simulink model "PMSMDriveThermal"  (R2025b)
settings: Solver=ode15s  StartTime=0.0  StopTime=1  MaxStep=1e-3  MinStep=1e-10  RelTol=1e-2  AbsTol=1e-6  EnableMultiTasking=on
PreLoadFcn:
  | PMSMDriveThermalData;
values from neighbouring files (symbols this model uses):
  N = 6    [E25runs1.mat]
  PM = 0.03    [E25runs1.mat]
undefined symbols (not defined in the file or in its folder): f_losses, Isc_losses, losses_oc, losses_sc
libraries: batteryecm_lib x280, fl_lib x53, nesl_utility x21, ee_lib x10, SimscapeFluids_lib x3, eePmsmFieldOrientedControl x1
(part 1 of 24)
CloseFcn:
  | try,close(h1_PMSMDriveThermal),end
  | clear h1_PMSMDriveThermal
  | try,close(h2_PMSMDriveThermal),end
  | clear h2_PMSMDriveThermal
  | 
  | clear simlog_PMSMDriveThermal
  | clear logsout_PMSMDriveThermal
  | 
  | clear alpha alpha_flux f_losses fc fnom fsw Imax
  | clear Isc losses J L0 Ld losses_oc losses_sc Lq N
  | clear omegam_nom PM Pmax rpm_nom Rs
  | clear Rd_percent_rotor Rm_percent_rotor
  | clear rotor_thermal_mass stator_thermal_mass
  | clear Tmax Tmeas Ts Tsc Isc_losses
Description:
  | Three-Phase PMSM Drive with Thermal Model
settings Model: Creator=The MathWorks, Inc.  LastModifiedBy=muizz
settings SolverCC: AutoScaleAbsTol=off  InitialStep=1e-8  MaxConsecutiveMinStep=20  ZeroCrossAlgorithm=Adaptive  AlgebraicLoopSolver=TrustRegion  MaxZcPerStep=1.0
settings DataIOCC: LimitDataPoints=on  MaxDataPoints=690000  SaveFormat=Array  ReturnWorkspaceOutputs=off  SignalLoggingName=logsout_PMSMDriveThermal
settings OptimizationCC: ReuseModelBlockBuffer=off  LifeSpan=inf
settings DebuggingCC: UnderspecifiedInitializationDetection=Classic  MergeDetectMultiDrivingBlocksExec=none  MaxConsecutiveZCsMsg=none  IgnoredZcDiagnostic=none  UnconnectedInputMsg=warning  UnconnectedOutputMsg=warning  UnconnectedLineMsg=warning  AllowSymbolicDim=off  PregeneratedLibrarySubsystemCodeDiagnostic=none  SFUnexpectedBacktrackingDiag=warning  SFNoUnconditionalDefaultTransitionDiag=warning  SFExecutionAtInitializationDiag=none  ArithmeticOperatorsInVariantConditions=warning
settings HardwareCC: ProdBitPerPointer=32.0  ProdBitPerSizeT=32.0  ProdBitPerPtrDiffT=32.0  ProdLargestAtomicFloat=None  ProdIntDivRoundTo=Undefined  ProdEndianess=Unspecified  ProdWordSize=32.0  ProdHWDeviceType=32-bit Generic
settings ModelReferenceCC: EnableRefExpFcnMdlSchedulingChecks=on  PropagateSignalLabelsOutOfModel=off
settings SFSimCC: SimUseLocalCustomCode=off
settings RTWCC: RTWUseLocalCustomCode=off  GPUComputeCapability=3.5  DLArmComputeVersion=19.05
settings CodeAppCC: StateflowObjectComments=on
settings GRTTargetCC: TargetLangStandard=C89/C90 (ANSI)
settings ConfigComp: CovMetricSettings=dw  CovSaveCumulativeToWorkspaceVar=on  CovSaveSingleToWorkspaceVar=on  CovExternalEMLEnable=off  CovSFcnEnable=off
settings SimscapeCC: SimscapeLogType=all  SimscapeLogSimulationStatistics=on  SimscapeLogName=simlog_PMSMDriveThermal  SimscapeLogDataHistory=690000.0

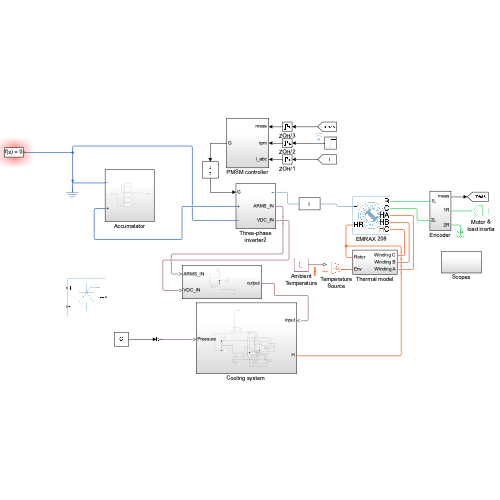
[thumbnail: Simulink's stored preview of the top-level diagram]
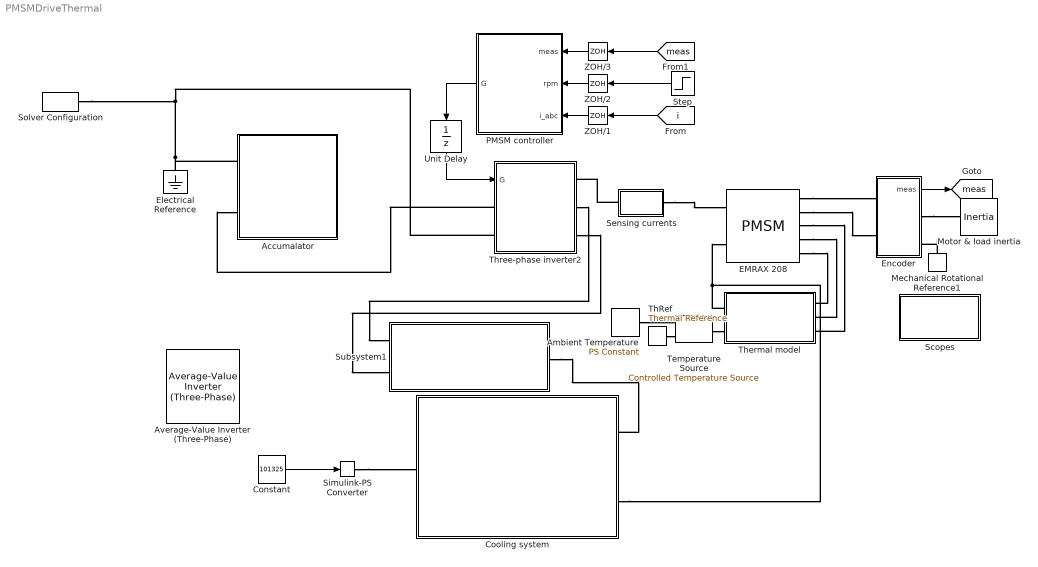
== system PMSMDriveThermal ==
  Accumalator : Subsystem
  Ambient Temperature : fl_lib/Physical Signals/Sources/PS Constant  constant=300.15 K
  Average-Value Inverter (Three-Phase) : ee_lib/Semiconductors & Converters/Converters/Average-Value Inverter (Three-Phase)  port_option=ee.enum.threePhasePort.composite  FRated=60 Hz  PhaseShift=0 deg  voltage_ratio=sqrt(6) / pi  Pfixed=1e3 W  v_on=100 V  v_off=75 V
      settings: InternalSimscapePortConfiguration="{\"Bottom\":[],\"Left\":[{\"id\":\"p\",\"label\":\"+\",\"type\":\"foundation.electrical.electrical\"},{\"id\":\"n\",\"label\":\"-\",\"type\":\"foundation.electrical.electrical\"}],\"Right\":[{\"id\":\"N\",\"label\":\"~\",\"type\":\"foundation.electrical.three_phase\"}],\"Top\":[]}"
  Constant : Constant  Value=101325
  "Cooling system " : Subsystem
  EMRAX 208 : ee_lib/Electromechanical/Permanent Magnet/PMSM  port_option=ee.enum.threePhasePort.composite  winding_type=ee.enum.electromech.statorconfiguration.wye  machine_param=ee.enum.pmsm.parameterization.constant  nPolePairs=10  pmflux_param=ee.enum.pmflux.fluxlinkage  pm_flux_linkage=0.23 Wb  torque_constant=0.916923438250803 % Datasheet derived N*m/A  back_emf_constant=0.916923438250803 % Datasheet derived V/(rad/s)  stator_param=ee.enum.statorparam.LdLqL0  Ld=0.138 mH  Lq=0.138 mH  idVec=[-200, 0, 200] A  iqVec=[-200, 0, 200] A  LdMatrix=0.0002 * ones(3, 3) H  LqMatrix=0.0002 * ones(3, 3) H  PmMatrix=0.1 * ones(3, 3) Wb  ktMatrix=0.18 * ones(3, 3) N*m/A  keMatrix=0.18 * ones(3, 3) V*s/rad  L0=0.00016 H  Ls=0.0002 H  Lm=-0.00002 H  Ms=0.00002 H  Rs=12 mOhm  zero_sequence=ee.enum.park.zerosequence.exclude  axes_param=ee.enum.rotorangle.daxis  loss_param=ee.enum.ironloss.none  losses_oc=[0, 0, 0] W  losses_sc=[0, 0, 0] W  f_losses=60 Hz  Isc_losses=95 A  J=256 kg*cm^2  lam=0 N*m*s/rad  i_d_specify=off  i_d_priority=None  i_d=0 A  i_d_nominal_specify=off  i_d_nominal_value=1  i_d_nominal_unit=A  i_q_specify=off  i_q_priority=None  i_q=0 A  i_q_nominal_specify=off  i_q_nominal_value=1  i_q_nominal_unit=A  torque_specify=off  torque_priority=High  torque=80 N*m  torque_nominal_specify=on  torque_nominal_value=80  torque_nominal_unit=N*m  angular_velocity_specify=off  angular_velocity_priority=High  angular_velocity=0 rpm  angular_velocity_nominal_specify=off  angular_velocity_nominal_value=1  angular_velocity_nominal_unit=rpm  angular_position_specify=off  angular_position_priority=High  angular_position=0 deg  angular_position_nominal_specify=off  angular_position_nominal_value=1  angular_position_nominal_unit=deg  alpha=3.93e-3 1/K  alpha_flux=-0.001 1/K  Tmeas=298.15 K  stator_thermal_mass=423.5 J/K  rotor_thermal_mass=2714 J/K  Rm_percent_rotor=90  Rd_percent_rotor=30  temperatureA_specify=off  temperatureA_priority=High  temperatureA=25 degC  temperatureA_nominal_specify=off  temperatureA_nominal_value=1  temperatureA_nominal_unit=degC  temperatureB_specify=off  temperatureB_priority=High  temperatureB=25 degC  temperatureB_nominal_specify=off  temperatureB_nominal_value=1  temperatureB_nominal_unit=degC  temperatureC_specify=off  temperatureC_priority=High  temperatureC=25 degC  temperatureC_nominal_specify=off  temperatureC_nominal_value=1  temperatureC_nominal_unit=degC  temperatureR_specify=off  temperatureR_priority=High  temperatureR=25 degC  temperatureR_nominal_specify=off  temperatureR_nominal_value=1  temperatureR_nominal_unit=degC
      settings: InternalSimscapePortConfiguration="{\"Bottom\":[],\"Left\":[{\"id\":\"N\",\"label\":\"~\",\"type\":\"foundation.electrical.three_phase\"},{\"id\":\"HR\",\"label\":\"HR\",\"type\":\"foundation.thermal.thermal\"}],\"Right\":[{\"id\":\"R\",\"label\":\"R\",\"type\":\"foundation.mechanical.rotational.rotational\"},{\"id\":\"C\",\"label\":\"C\",\"type\":\"foundation.mechanical.rotational.rotational\"},{\"id\":\"HA\",\"label\":\"HA\",\"type\":\"foundation.thermal.thermal\"},{\"id\":\"HB\",\"label\":\"HB\",\"type\":\"foundation.thermal.thermal\"},{\"id\":\"HC\",\"label\":\"HC\",\"type\":\"foundation.thermal.thermal\"}],\"Top\":[]}"
  Electrical Reference : fl_lib/Electrical/Electrical Elements/Electrical Reference
  Encoder : Subsystem
  Mechanical Rotational Reference1 : fl_lib/Mechanical/Rotational Elements/Mechanical Rotational Reference
  Motor & load inertia : fl_lib/Mechanical/Rotational Elements/Inertia  inertia=256 kg*m^2  num_ports=foundation.enum.numPorts2.one  w_specify=on  w_priority=High  w=0 rpm  w_nominal_specify=off  w_nominal_value=1  w_nominal_unit=rad/s  t_specify=off  t_priority=High  t=0 N*m  t_nominal_specify=off  t_nominal_value=1  t_nominal_unit=N*m
  PMSM controller : Subsystem
  Scopes : Subsystem
  Sensing currents : Subsystem
      mask Display: disp('i')
  Simulink-PS Converter : nesl_utility/Simulink-PS Converter  PhysicalDomain=network_engine_domain  SubClassName=ps_input  LeftPortType=input  RightPortType=output  PseudoPeriodic=off  Frequencies=[]  NoiseDistribution=none  NoiseParameters=[]  Unit=1  AffineConversion=off  FilteringAndDerivatives=provide  SimscapeFilterOrder=1  InputFilterTimeConstant=0.001  UdotUserProvided=0
  Solver Configuration : nesl_utility/Solver Configuration  PhysicalDomain=network_engine_domain  SubClassName=solver  LeftPortType=input  RightPortType=generic  Tones=[]  Harmonics=[]  SimulateNoise=off  Profile=off  UseLocalSampling=off  EnableSwitchedLinearOptims=on  FrequencyDomain=off  UseCCode=off  RelTol=0.001  AbsTol=1e-06  MinStep=1e-09  ToWorkspace=off  RevertToSquareIcSolve=off  NumHomotopyIterations=100  PhasorMode=off  PhasorModeNumHarmonics=1  ConsistencySolver=NEWTON_FTOL  IndexReductionMethod=DerivativeReplacement  DoDC=off  ResidualTolerance=1e-3  ConsistencyTolSource=GLOBAL  ConsistencyAbsTol=0.001  ConsistencyRelTol=0.001  ConsistencyTolFactor=0.001  UseLocalSolver=off  LocalSolverChoice=NE_BACKWARD_EULER_ADVANCER  ResolveIndetEquations=on  FunctionEvalNumThread=1  LocalSolverSampleTime=Ts  DoFixedCost=on  MaxNonlinIter=6  MaxModeIter=2  ComputeImpulses=off  ImpulseIterations=2  LinearAlgebra=auto  LinearAlgebraNumThread=0  EquationFormulation=NE_TIME_EF  DelaysMemoryBudget=1024  AutomaticFiltering=on  FilteringTimeConstant=0.001  PartitionStorageMethod=AS_NEEDED  PartitionMemoryBudget=1024  PartitionMethod=FAST  MultibodyUseLocalSolver=off  MultibodyLocalSolverChoice=ODE1  MultibodyLocalSolverSampleTime=0.001
  Step : Step  Time=0.1  After=500  SampleTime=0
  Subsystem1 : Subsystem
  Temperature Source : fl_lib/Thermal/Thermal Sources/Controlled Temperature Source
  ThRef : fl_lib/Thermal/Thermal Elements/Thermal Reference
  Thermal model : Subsystem  Tag=PublishSubsystem
  Three-phase inverter2 : Subsystem
  Unit Delay : UnitDelay  SampleTime=-1  HasFrameUpgradeWarning=on
  ZOH/1 : ZeroOrderHold  SampleTime=2e-05
  ZOH/2 : ZeroOrderHold  SampleTime=2e-05
  ZOH/3 : ZeroOrderHold  SampleTime=2e-05
  tag scope: meas=global
  wires:
  Step/1 -> ZOH/2/1
  ZOH/3/1 -> PMSM controller/1(meas)
  ZOH/2/1 -> PMSM controller/2(rpm)
  ZOH/1/1 -> PMSM controller/3(i_abc)
  PMSM controller/1(G) -> Unit Delay/1
  [i] -> ZOH/1/1
  Encoder/1(meas) -> [meas]
  [meas] -> ZOH/3/1
  Constant/1 -> Simulink-PS Converter/1
  Unit Delay/1 -> Three-phase inverter2/1(G)
  connections:
  EMRAX 208/RConn1 -- Encoder/LConn1
  EMRAX 208/RConn2 -- Encoder/LConn2
  Encoder/RConn1 -- Motor & load inertia/LConn1
  Mechanical Rotational Reference1/LConn1 -- Encoder/RConn2
  Electrical Reference/LConn1 -- Accumalator/LConn1 -- Three-phase inverter2/LConn2 -- Solver Configuration/RConn1
  EMRAX 208/RConn5 -- Thermal model/RConn1
  Ambient Temperature/RConn1 -- Temperature Source/RConn1
  ThRef/LConn1 -- Temperature Source/RConn2
  EMRAX 208/RConn3 -- Thermal model/RConn3
  EMRAX 208/RConn4 -- Thermal model/RConn2
  Temperature Source/LConn1 -- Thermal model/LConn2
  Thermal model/LConn1 -- EMRAX 208/LConn2 -- "Cooling system "/RConn2
  Sensing currents/RConn1 -- EMRAX 208/LConn1
  Three-phase inverter2/LConn1 -- Accumalator/LConn2
  Sensing currents/LConn1 -- Three-phase inverter2/RConn1
  Three-phase inverter2/RConn2 -- Subsystem1/LConn1
  Three-phase inverter2/RConn3 -- Subsystem1/LConn2
  Simulink-PS Converter/RConn1 -- "Cooling system "/LConn1
  Subsystem1/RConn1 -- "Cooling system "/RConn1

== system PMSMDriveThermal/Accumalator ==
  Module  four : Subsystem
  Module Five1 : Subsystem
  Module One1 : Subsystem
  Module Three1 : Subsystem
  "Module Two " : Subsystem
  - : PMIOPort  Side=Left
  + : PMIOPort  Port=2  Side=Left
  connections:
  "Module Two "/LConn2 -- Module Three1/LConn1
  Module Three1/LConn2 -- Module  four/LConn1
  Module One1/LConn2 -- "Module Two "/LConn1
  Module  four/LConn2 -- Module Five1/LConn1
  Module Five1/LConn2 -- -/RConn1
  Module One1/LConn1 -- +/RConn1
